simulink model "TestMotionLaw"  (R2021b)
settings: Solver=VariableStepAuto  StartTime=0.0  StopTime=500  RelTol=1e-3
values from neighbouring files (symbols this model uses):
  floor_height = 3    [test_LiftDynamicsEquation.m]    (also in test_discretization.m)
  Ts = 1e-3    (= 0.001)    [test_LiftDynamicsEquation.m]    (also in test_discretization.m; test_motion_law.m = 0.01)
undefined symbols (not defined in the file or in its folder): num_floor
settings Model: Creator=manue  LastModifiedBy=manue

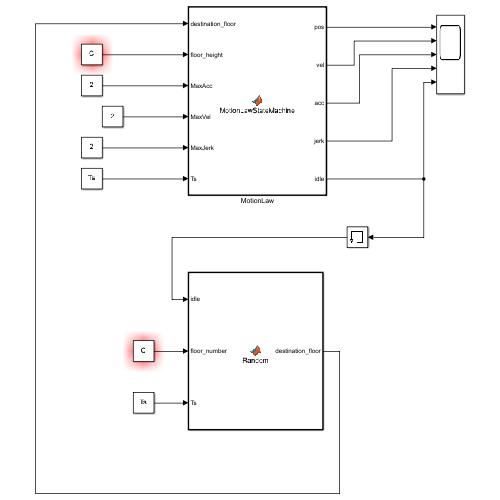
[thumbnail: Simulink's stored preview of the top-level diagram]
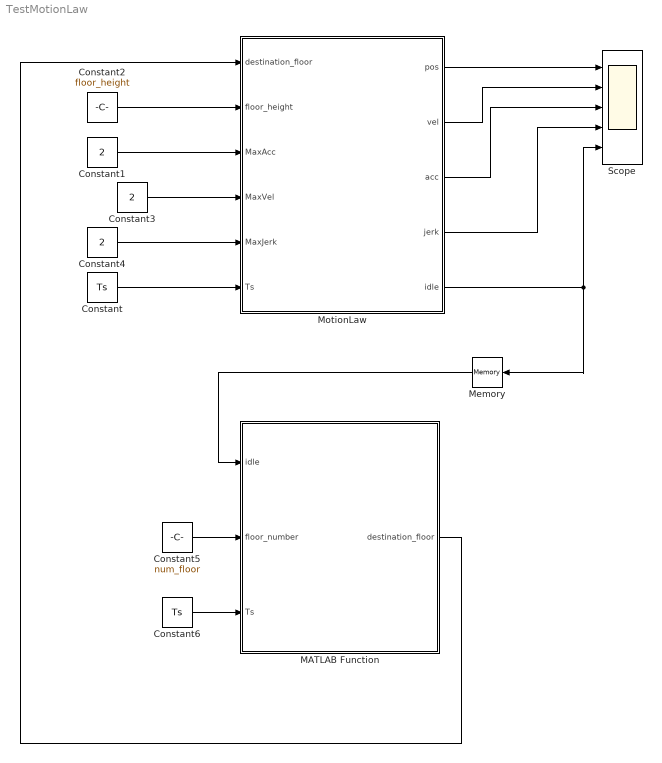
== system TestMotionLaw ==
  Constant : Constant  Value=Ts
  Constant1 : Constant  Value=2
  Constant2 : Constant  Value=floor_height
  Constant3 : Constant  Value=2
  Constant4 : Constant  Value=2
  Constant5 : Constant  Value=num_floor
  Constant6 : Constant  Value=Ts
  MATLAB Function : MATLAB Function  TreatAsAtomicUnit=on  SystemSampleTime=Ts
  Memory : Memory
  MotionLaw : MATLAB Function  TreatAsAtomicUnit=on  SystemSampleTime=Ts
  Scope : Scope  NumInputPorts=5
  wires:
  Constant/1 -> MotionLaw/6(Ts)
  Constant1/1 -> MotionLaw/3(MaxAcc)
  Constant2/1 -> MotionLaw/2(floor_height)
  MotionLaw/1(pos) -> Scope/1
  MotionLaw/5(idle) -> Memory/1, Scope/5
  Constant4/1 -> MotionLaw/5(MaxJerk)
  Constant3/1 -> MotionLaw/4(MaxVel)
  MotionLaw/2(vel) -> Scope/2
  MotionLaw/3(acc) -> Scope/3
  MotionLaw/4(jerk) -> Scope/4
  Constant6/1 -> MATLAB Function/3(Ts)
  Constant5/1 -> MATLAB Function/2(floor_number)
  MATLAB Function/1(destination_floor) -> MotionLaw/1(destination_floor)
  Memory/1 -> MATLAB Function/1(idle)

== matlab function TestMotionLaw/MotionLaw ==
  data: destination_floor input; floor_height input; MaxAcc input; MaxVel input; MaxJerk input; Ts input; pos output; vel output; acc output; jerk output; idle output
function [pos,vel,acc,jerk,idle]  = MotionLawStateMachine(destination_floor,floor_height,MaxAcc,MaxVel,MaxJerk,Ts)

persistent state last_floor time duration direction t1 t2 t4 destination_floor_
if isempty(state)
    state=0; %IDLE
    last_floor=destination_floor;
    destination_floor_=destination_floor;
    time=0;
    duration=1;
    direction=0;
    t1=0;
    t2=0;
    t4=0;

end


idle=false;


if (state==0) && (destination_floor~=last_floor)
    state=1; % TRANSITION
    time=0;
    CruiseVel=MaxVel;
    destination_floor_=destination_floor;
    distance=abs(destination_floor-last_floor)*floor_height;


    direction=sign(destination_floor-last_floor);


    if MaxVel>MaxAcc^2/(2*MaxJerk)
        %case 1
        limit_distance_case1=(MaxVel*(MaxAcc^2 + MaxVel*MaxJerk))/(MaxAcc*MaxJerk);


        if (distance>limit_distance_case1)
            % case 1.1
            CruiseVel=MaxVel;
            law_case=11;
        else
            CruiseVel=-(MaxAcc^2 - MaxAcc^(1/2)*(MaxAcc^3 + 4*distance*MaxJerk^2)^(1/2))/(2*MaxJerk);

            if CruiseVel>MaxAcc^2/(2*MaxJerk)
                %case 1.2
                law_case=12;
            else
                limit_distance_case2=(2*CruiseVel^(3/2))/MaxJerk^(1/2);
                if distance>limit_distance_case2
                    law_case=21;
                else
                    law_case=22;
                end
            end
        end

    else
        limit_distance_case2=(2*MaxVel^(3/2))/MaxJerk^(1/2);
        if distance>limit_distance_case2
            law_case=21;
        else
            law_case=22;
        end
    end

    switch law_case
        case 11
            t1=MaxAcc/MaxJerk;
            t2=(- MaxAcc^2/MaxJerk + MaxVel)/MaxAcc;
            t4=(distance - (MaxVel*(MaxAcc^2 + MaxVel*MaxJerk))/(MaxAcc*MaxJerk))/MaxVel;
            CruiseVel=MaxVel;
        case 12
            t1=MaxAcc/MaxJerk;
            CruiseVel=-(MaxAcc^2 - MaxAcc^(1/2)*(MaxAcc^3 + 4*distance*MaxJerk^2)^(1/2))/(2*MaxJerk);
            t2=-(3*MaxAcc^(3/2) - (MaxAcc^3 + 4*distance*MaxJerk^2)^(1/2))/(2*MaxAcc^(1/2)*MaxJerk);
            t4=0;
        case 21
            %CruiseVel=MaxVel;
            t1=CruiseVel^(1/2)/MaxJerk^(1/2);
            t2=0;
            t4=(distance - (2*CruiseVel^(3/2))/MaxJerk^(1/2))/CruiseVel;

        otherwise % case 22
            CruiseVel=((MaxJerk^(1/2)*distance)/2)^(2/3);
            t1=CruiseVel^(1/2)/MaxJerk^(1/2);
            t2=0;
            t4=0;
    end
    duration=4*t1+2*t2+t4; % t1+t2+t3+t4+t5+t6+t7, t1=t3=t5=t6,t2=t6
elseif (state==1) && (time>=duration)
    state=0;
    last_floor=destination_floor_;
end

if (state==0)
    
    idle=true;
    pos=last_floor*floor_height;
    vel=0;
    acc=0;
    jerk=0;
else%if (state==1)
    time=time+Ts;
    [jerk,acc,vel,pos]=JerkMotionLaw(MaxJerk,t1,t2,t4,time)   ;
    if direction>0
        pos=last_floor*floor_height+pos;
    else
        pos=last_floor*floor_height-pos;
        vel=-vel;
        acc=-acc;
        jerk=-jerk;
    end
    idle=false;
end

end

function [jerk,acc,vel,pos]=JerkMotionLaw(MaxJerk,t1,t2,t4,time)   

if (time<t1)
	jerk=MaxJerk;
	acc=MaxJerk*time;
	vel=(MaxJerk*time^2)/2;
	pos=(MaxJerk*time^3)/6;
elseif (time<t1 + t2)
	jerk=0;
	acc=MaxJerk*t1;
	vel=(MaxJerk*t1^2)/2 - MaxJerk*t1*(t1 - time);
	pos=(MaxJerk*t1^3)/6 - (MaxJerk*t1*time*(t1 - time))/2;
elseif (time<2*t1 + t2)
	jerk=-MaxJerk;
	acc=MaxJerk*t1 + MaxJerk*(t1 + t2 - time);
	vel=(MaxJerk*t1*(t1 + 2*t2))/2 - (MaxJerk*(4*t1*t2 - 4*t1*time - 2*t2*time + 3*t1^2 + t2^2 + time^2))/2;
	pos=(MaxJerk*t1^3)/6 - (MaxJerk*(t1 + t2 - time)*(t1*t2 + 5*t1*time + 2*t2*time - t1^2 - t2^2 - time^2))/6 + (MaxJerk*t1*t2*(t1 + t2))/2;
elseif (time<2*t1 + t2 + t4)
	jerk=0;
	acc=0;
	vel=MaxJerk*t1*(t1 + t2);
	pos=(MaxJerk*t1*(3*t1*t2 + 2*t1^2 + t2^2))/2 - MaxJerk*t1*(t1 + t2)*(2*t1 + t2 - time);
elseif (time<3*t1 + t2 + t4)
	jerk=-MaxJerk;
	acc=MaxJerk*(2*t1 + t2 + t4 - time);
	vel=MaxJerk*t1*(t1 + t2) - (MaxJerk*(2*t1 + t2 + t4 - time)^2)/2;
	pos=(MaxJerk*t1*(t1 + t2)*(2*t1 + t2 + 2*t4))/2 - (MaxJerk*(2*t1 + t2 + t4 - time)*(2*t1*t2 - 4*t1*t4 - 2*t2*t4 + 4*t1*time + 2*t2*time + 2*t4*time + 2*t1^2 - t2^2 - t4^2 - time^2))/6;
elseif (time<3*t1 + 2*t2 + t4)
	jerk=0;
	acc=-MaxJerk*t1;
	vel=MaxJerk*t1*(3*t1 + t2 + t4 - time) + (MaxJerk*t1*(t1 + 2*t2))/2;
	pos=(MaxJerk*t1*(15*t1*t2 + 6*t1*t4 + 6*t2*t4 + 11*t1^2 + 3*t2^2))/6 - (MaxJerk*t1*(13*t1*t2 + 7*t1*t4 + 4*t2*t4 - 7*t1*time - 4*t2*time - 2*t4*time + 12*t1^2 + 3*t2^2 + t4^2 + time^2))/2;
elseif (time<4*t1 + 2*t2 + t4)
	jerk=MaxJerk;
	acc=- MaxJerk*t1 - MaxJerk*(3*t1 + 2*t2 + t4 - time);
	vel=(MaxJerk*t1^2)/2 + (MaxJerk*(16*t1*t2 + 8*t1*t4 + 4*t2*t4 - 8*t1*time - 4*t2*time - 2*t4*time + 15*t1^2 + 4*t2^2 + t4^2 + time^2))/2;
	pos=(MaxJerk*t1*(18*t1*t2 + 6*t1*t4 + 6*t2*t4 + 11*t1^2 + 6*t2^2))/6 - (MaxJerk*(48*t1*t2^2 + 96*t1^2*t2 + 12*t1*t4^2 + 48*t1^2*t4 + 6*t2*t4^2 + 12*t2^2*t4 + 12*t1*time^2 - 48*t1^2*time + 6*t2*time^2 - 12*t2^2*time + 3*t4*time^2 - 3*t4^2*time + 63*t1^3 + 8*t2^3 + t4^3 - time^3 + 48*t1*t2*t4 - 48*t1*t2*time - 24*t1*t4*time - 12*t2*t4*time))/6;
else
	jerk=0;
	acc=0;
	vel=0;
	pos=MaxJerk*t1*(t1 + t2)*(2*t1 + t2 + t4);
end
end

== matlab function TestMotionLaw/MATLAB Function ==
  data: idle input; destination_floor output; floor_number input; Ts input
function destination_floor = Random(idle,floor_number,Ts)

persistent destination_floor_ state time wait_time;
if isempty(destination_floor_)
    destination_floor_=0;
    state=0;
    time=0;
    wait_time=0;
end

if (state==0 && idle) % wait a random time
    wait_time=5+5*rand();
    time=0;
    state=1;
elseif (state==1 && time>wait_time)
    state=2;
elseif (state==2)
    state=0;
end

time=time+Ts;
if (state==2)
    destination_floor_=randi(floor_number);
end

destination_floor=destination_floor_;
